simulink model "Simulation_BlackBox"  (R2022b)
settings: Solver=VariableStepAuto  StartTime=0.0  StopTime=100  RelTol=1e-3
undefined symbols (not defined in the file): DiscIntNeverNeededParam, drv, gbox, mot, sens, Tc, Ts
settings Model: Creator=Matteo  LastModifiedBy=david
settings SolverCC: AlgebraicLoopSolver=LineSearch
settings DebuggingCC: UnconnectedInputMsg=warning  UnconnectedOutputMsg=warning  UnconnectedLineMsg=warning  SFMachineParentedDataDiag=warning  ArithmeticOperatorsInVariantConditions=warning
settings ModelReferenceCC: EnableRefExpFcnMdlSchedulingChecks=on
settings SFSimCC: SimUseLocalCustomCode=off  CustomCodeUndefinedFunction=UseInterfaceOnly
settings RTWCC: RTWUseLocalCustomCode=off

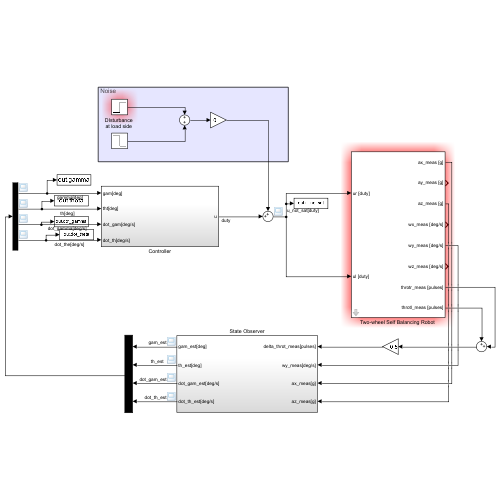
[thumbnail: Simulink's stored preview of the top-level diagram]
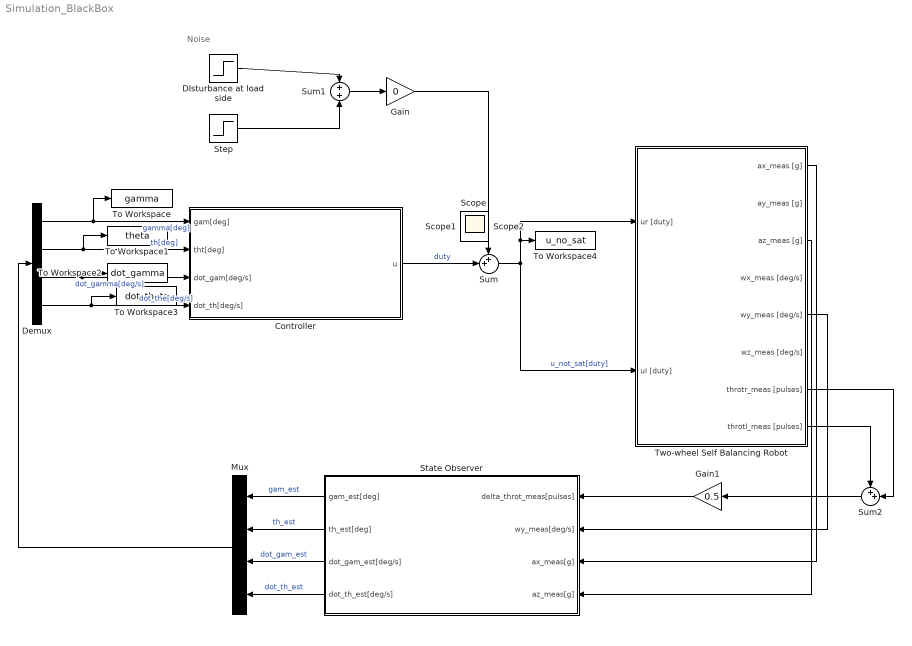
== system Simulation_BlackBox ==
  note: Noise
  Controller : Subsystem
  "DIsturbance at load side " : Step  Time=30  After=100  SampleTime=Ts
  Demux : Demux
  Gain : Gain  Gain=0
  Gain1 : Gain  Gain=0.5
  Mux : Mux
  State Observer : Subsystem
  Step : Step  Time=60  After=-100  SampleTime=0
  Sum : Sum  Inputs=++|
  Sum1 : Sum
  Sum2 : Sum  Inputs=++|
  To Workspace : ToWorkspace  VariableName=gamma  SaveFormat=Structure With Time  SampleTime=0.01
  To Workspace1 : ToWorkspace  VariableName=theta  SaveFormat=Structure With Time  SampleTime=0.01
  To Workspace2 : ToWorkspace  VariableName=dot_gamma  SaveFormat=Structure With Time  SampleTime=0.01
  To Workspace3 : ToWorkspace  VariableName=dot_theta  SaveFormat=Structure With Time  SampleTime=0.01
  To Workspace4 : ToWorkspace  VariableName=u_no_sat  SaveFormat=Structure With Time  SampleTime=0.01
  "Two-wheel Self Balancing Robot " : Subsystem  mask(Balancing robot (longitudinal + lateral dynamics)){initState=[0, 0, pi/36, 0, 0, 0], Ts=Ts}
      mask prompts: initState "Initial state [gam(0), psi(0), th(0), dot_gam(0), dot_psi(0), dot_th(0)]'"; Ts "Sample time:"
      mask help:
      | Balancing robot dynamic model.
      | Includes both the longitudinal and lateral (yaw) dynamics.
      mask init:
      | %% General parameters and conversion gains
      | 
      | %   gravity acc [m/s^2]
      | g = 9.81;
      | 
      | %   conversion gains
      | rpm2rads = 2*pi/60;         %   [rpm]   -> [rad/s]
      | rads2rpm = 60/2/pi;         %   [rad/s] -> [rpm]
      | rpm2degs = 360/60;          %   [rpm]   -> [deg/s]
      | degs2rpm = 60/360;          %   [deg/s] -> [rpm]
      | deg2rad = pi/180;           %   [deg]   -> [rad]
      | rad2deg = 180/pi;           %   [rad]   -> [deg]
      | g2ms2 = g;                  %   [acc_g] -> [m/s^2]
      | ms22g = 1/g;                %   [m/s^2] -> [acc_g]
      | ozin2Nm = 0.706e-2;         %   [oz*inch] -> [N*m]
      | 
      | 
      | %%  Battery data
      | 
      | %   electrical data
      | batt.UN = 11.1;     %   nominal voltage
      | 
      | 
      | %%  H-bridge PWM voltage driver
      | 
      | drv.Vbus = batt.UN;                     %   H-bridge DC bus voltage  
      | drv.pwm.bits = 8;                       %   PWM resolution [bits]
      | drv.pwm.levels = 2^drv.pwm.bits;        %   PWM levels
      | drv.pwm.Fs = 490;                       %   PWM frequency
      | drv.dutymax = drv.pwm.levels-1;         %   max duty cycle code
      | drv.duty2V = drv.Vbus/drv.dutymax;      %   duty cycle code (0-255) to voltage
      | drv.V2duty = drv.dutymax/drv.Vbus;      %   voltage to duty cycle code (0-255)
      | 
      | 
      | %%  Gearbox data 
      | 
      | gbox.N = 30;            %   reduction ratio
      | 
      | 
      | %%  Sensors data - Hall-effect encoder
      | 
      | %   Hall-effect encoder
      | sens.enc.ppr = 16*4;    %   pulses per rotation at motor side (w/ quadrature decoding)
      | sens.enc.pulse2deg = 360/sens.enc.ppr;
      | sens.enc.pulse2rad = 2*pi/sens.enc.ppr;
      | sens.enc.deg2pulse = sens.enc.ppr/360;
      | sens.enc.rad2pulse = sens.enc.ppr/2/pi;
      | 
      | 
      | %%  Sensors data - MPU6050 (accelerometer + gyro)
      | 
      | %   center of mass (CoM) position
      | sens.mpu.xb = 0;
      | sens.mpu.yb = 0;
      | sens.mpu.zb = 13.5e-3;
      | 
      | %       MPU6050 embedded accelerometer specs
      | sens.mpu.acc.bits = 16;
      | sens.mpu.acc.fs_g = 16;                                                         %   full-scale in "g" units
      | sens.mpu.acc.fs = sens.mpu.acc.fs_g * g2ms2;                                    %   full-scale in [m/s^2] 
      | sens.mpu.acc.g2LSB = floor(2^(sens.mpu.acc.bits-1)/sens.mpu.acc.fs_g);          %   sensitivity [LSB/g]
      | sens.mpu.acc.ms22LSB = sens.mpu.acc.g2LSB * ms22g;                              %   sensitvity [LSB/(m/s^2)]
      | sens.mpu.acc.LSB2g = sens.mpu.acc.fs_g/2^(sens.mpu.acc.bits-1);                 %   output quantization step [g/LSB]
      | sens.mpu.acc.LSB2ms2 = sens.mpu.acc.LSB2g * g2ms2;                              %   output quantization step [ms2/LSB]
      | sens.mpu.acc.bw = 94;                                                           %   output low-pass filter bandwidth
      | sens.mpu.acc.noisestd = 400e-6*sqrt(100);                                       %   output noise std [g-rms]
      | sens.mpu.acc.noisevar = sens.mpu.acc.noisestd^2;                                %   output noise var [g^2]
      | 
      | %       MPU6050 embdedded gyroscope specs
      | sens.mpu.gyro.bits = 16;
      | sens.mpu.gyro.fs_degs = 250;                                                    %   full scale in [deg/s (dps)]
      | sens.mpu.gyro.fs = sens.mpu.gyro.fs_degs * deg2rad;                             %   full scale in [rad/s]
      | sens.mpu.gyro.degs2LSB = floor(2^(sens.mpu.gyro.bits-1)/sens.mpu.gyro.fs_degs);	%   sensitivity [LSB/degs]
      | sens.mpu.gyro.rads2LSB = sens.mpu.gyro.degs2LSB * rad2deg;                      %   sensitivity [LSB/rads] 
      | sens.mpu.gyro.LSB2degs = sens.mpu.gyro.fs_degs/2^(sens.mpu.gyro.bits-1);        %   output quantization step [degs/LSB]
      | sens.mpu.gyro.LSB2rads = sens.mpu.gyro.LSB2degs * deg2rad;                      %   output quantization step [rads/LSB]
      | sens.mpu.gyro.bw = 98;                                                          %   output low-pass filter bandwidth
      | sens.mpu.gyro.noisestd = 5e-3*sqrt(100);                                        %   output noise std [degs-rms]
      | sens.mpu.gyro.noisevar = sens.mpu.acc.noisestd ^2;                              %   output noise var [degs^2]
      mask Help:
      | Riccardo Antonello (antonello@dei.unipd.it)
      | 
      | May 19, 2020
      | 
      | Dept. of Information Engineering, University of Padova
  Scope : Scope
  Scope1 : Scope
  Scope2 : Scope
  wires:
  "DIsturbance at load side "/1 -> Sum1/1
  Sum2/1 -> Gain1/1
  "Two-wheel Self Balancing Robot "/5(wy_meas [deg/s]) -> State Observer/2(wy_meas[deg/s])
  "Two-wheel Self Balancing Robot "/1(ax_meas [g]) -> State Observer/3(ax_meas[g])
  "Two-wheel Self Balancing Robot "/3(az_meas [g]) -> State Observer/4(az_meas[g])
  Sum/1 -> "Two-wheel Self Balancing Robot "/1(ur [duty]), To Workspace4/1, "Two-wheel Self Balancing Robot "/2(ul [duty])  "u_not_sat[duty]"
  Controller/1(u) -> Sum/2  "duty"
  Demux/3 -> To Workspace2/1, Controller/3(dot_gam[deg/s])  "dot_gamma[deg/s]"
  Demux/2 -> To Workspace1/1, Controller/2(tht[deg])  "th[deg]"
  Demux/1 -> To Workspace/1, Controller/1(gam[deg])  "gamma[deg]"
  Demux/4 -> To Workspace3/1, Controller/4(dot_th[deg/s])  "dot_the[deg/s]"
  State Observer/1(gam_est[deg]) -> Mux/1  "gam_est"
  State Observer/2(th_est[deg]) -> Mux/2  "th_est"
  State Observer/3(dot_gam_est[deg/s]) -> Mux/3  "dot_gam_est"
  State Observer/4(dot_th_est[deg/s]) -> Mux/4  "dot_th_est"
  Mux/1 -> Demux/1
  Sum1/1 -> Gain/1
  Step/1 -> Sum1/2
  Gain/1 -> Sum/1
  Gain1/1 -> State Observer/1(delta_throt_meas[pulses])
  "Two-wheel Self Balancing Robot "/7(throtr_meas [pulses]) -> Sum2/2
  "Two-wheel Self Balancing Robot "/8(throtl_meas [pulses]) -> Sum2/1

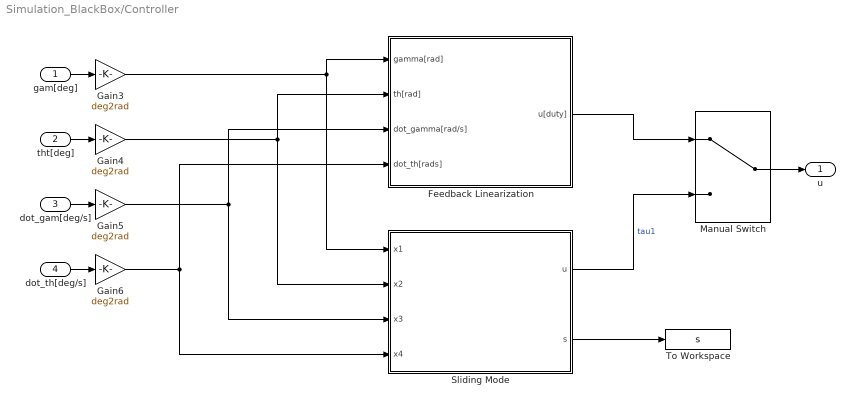
== system Simulation_BlackBox/Controller ==
  gam[deg] : Inport
  tht[deg] : Inport  Port=2
  dot_gam[deg/s] : Inport  Port=3
  dot_th[deg/s] : Inport  Port=4
  Feedback Linearization : Subsystem
  Gain{3..6} (4 alike) : Gain  Gain=deg2rad
  Manual Switch : ManualSwitch
  Sliding Mode : MATLAB Function  TreatAsAtomicUnit=on
  To Workspace : ToWorkspace  VariableName=s  SaveFormat=Structure With Time  SampleTime=0.01
  u : Outport  VectorParamsAs1DForOutWhenUnconnected=off
  wires:
  gam[deg]/1 -> Gain3/1
  dot_th[deg/s]/1 -> Gain6/1
  dot_gam[deg/s]/1 -> Gain5/1
  tht[deg]/1 -> Gain4/1
  Gain3/1 -> Feedback Linearization/1(gamma[rad]), Sliding Mode/1(x1)
  Gain4/1 -> Feedback Linearization/2(th[rad]), Sliding Mode/2(x2)
  Gain5/1 -> Feedback Linearization/3(dot_gamma[rad/s]), Sliding Mode/3(x3)
  Gain6/1 -> Feedback Linearization/4(dot_th[rads]), Sliding Mode/4(x4)
  Sliding Mode/1(u) -> Manual Switch/2  "tau1"
  Sliding Mode/2(s) -> To Workspace/1
  Manual Switch/1 -> u/1
  Feedback Linearization/1(u[duty]) -> Manual Switch/1

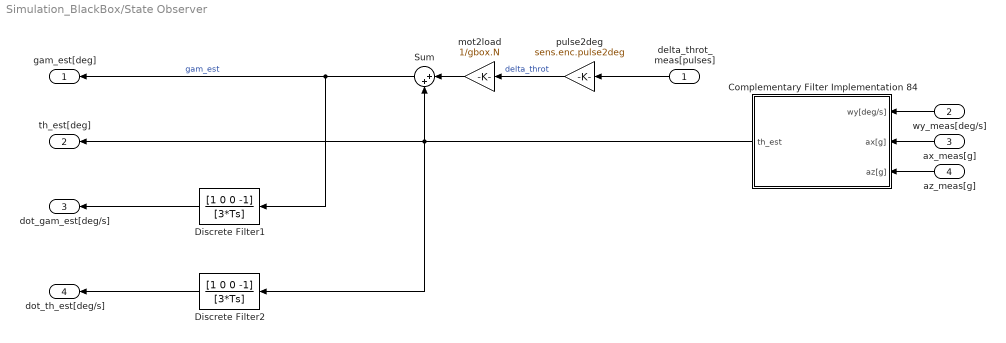
== system Simulation_BlackBox/State Observer ==
  delta_throt_meas[pulses] : Inport
  wy_meas[deg/s] : Inport  Port=2
  ax_meas[g] : Inport  Port=3
  az_meas[g] : Inport  Port=4
  Complementary Filter Implementation 84 : Subsystem
  Discrete Filter1 : DiscreteFilter  Numerator=[1 0 0 -1]  Denominator=[3*Ts]  SampleTime=Ts
  Discrete Filter2 : DiscreteFilter  Numerator=[1 0 0 -1]  Denominator=[3*Ts]  SampleTime=Ts
  Sum : Sum  Inputs=|++
  mot2load : Gain  Gain=1/gbox.N
  pulse2deg : Gain  Gain=sens.enc.pulse2deg
  gam_est[deg] : Outport  VectorParamsAs1DForOutWhenUnconnected=off
  th_est[deg] : Outport  Port=2  VectorParamsAs1DForOutWhenUnconnected=off
  dot_gam_est[deg/s] : Outport  Port=3  VectorParamsAs1DForOutWhenUnconnected=off
  dot_th_est[deg/s] : Outport  Port=4  VectorParamsAs1DForOutWhenUnconnected=off
  wires:
  Sum/1 -> Discrete Filter1/1, gam_est[deg]/1  "gam_est"
  Discrete Filter2/1 -> dot_th_est[deg/s]/1
  mot2load/1 -> Sum/1
  delta_throt_meas[pulses]/1 -> pulse2deg/1
  Complementary Filter Implementation 84/1(th_est) -> Discrete Filter2/1, th_est[deg]/1, Sum/2
  pulse2deg/1 -> mot2load/1  "delta_throt"
  Discrete Filter1/1 -> dot_gam_est[deg/s]/1
  az_meas[g]/1 -> Complementary Filter Implementation 84/3(az[g])
  ax_meas[g]/1 -> Complementary Filter Implementation 84/2(ax[g])
  wy_meas[deg/s]/1 -> Complementary Filter Implementation 84/1(wy[deg/s])

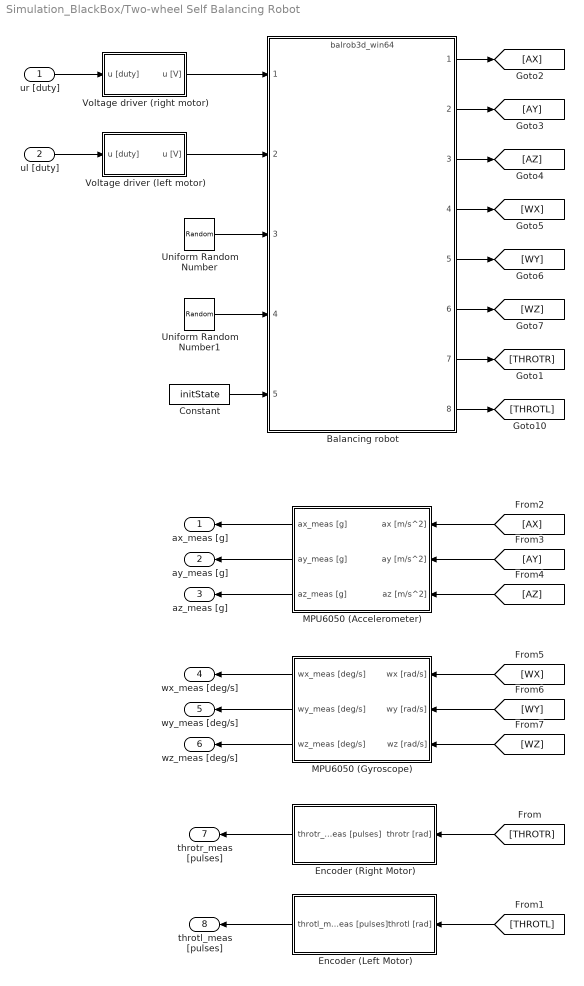
== system Simulation_BlackBox/Two-wheel Self Balancing Robot  ==
  ur [duty] : Inport
  ul [duty] : Inport  Port=2
  Balancing robot : ModelReference  ModelNameDialog=balrob3d_win64.slxp  ModelReferenceVersion=1.741  CopyOfModelProtected=on
  Constant : Constant  Value=initState
  Encoder (Left Motor) : Subsystem
  Encoder (Right Motor) : Subsystem
  MPU6050 (Accelerometer) : Subsystem
  MPU6050 (Gyroscope) : Subsystem
  Uniform Random Number : UniformRandomNumber  Minimum=0.7  Maximum=1.3  SampleTime=1
  Uniform Random Number1 : UniformRandomNumber  Minimum=0.7  Maximum=1.3  Seed=10  SampleTime=1
  Voltage driver (left motor) : Subsystem
  Voltage driver (right motor) : Subsystem
  ax_meas [g] : Outport
  ay_meas [g] : Outport  Port=2
  az_meas [g] : Outport  Port=3
  wx_meas [deg/s] : Outport  Port=4
  wy_meas [deg/s] : Outport  Port=5
  wz_meas [deg/s] : Outport  Port=6
  throtr_meas [pulses] : Outport  Port=7
  throtl_meas [pulses] : Outport  Port=8
  wires:
  ur [duty]/1 -> Voltage driver (right motor)/1(u [duty])
  [WX] -> MPU6050 (Gyroscope)/1(wx [rad/s])
  Balancing robot/2 -> [AY]
  Balancing robot/4 -> [WX]
  Balancing robot/8 -> [THROTL]
  Balancing robot/1 -> [AX]
  [THROTL] -> Encoder (Left Motor)/1(throtl [rad])
  Balancing robot/6 -> [WZ]
  Balancing robot/7 -> [THROTR]
  Balancing robot/5 -> [WY]
  [AX] -> MPU6050 (Accelerometer)/1(ax [m/s^2])
  [WY] -> MPU6050 (Gyroscope)/2(wy [rad/s])
  Balancing robot/3 -> [AZ]
  [WZ] -> MPU6050 (Gyroscope)/3(wz [rad/s])
  [AZ] -> MPU6050 (Accelerometer)/3(az [m/s^2])
  [THROTR] -> Encoder (Right Motor)/1(throtr [rad])
  ul [duty]/1 -> Voltage driver (left motor)/1(u [duty])
  [AY] -> MPU6050 (Accelerometer)/2(ay [m/s^2])
  MPU6050 (Accelerometer)/1(ax_meas [g]) -> ax_meas [g]/1
  MPU6050 (Accelerometer)/2(ay_meas [g]) -> ay_meas [g]/1
  MPU6050 (Accelerometer)/3(az_meas [g]) -> az_meas [g]/1
  MPU6050 (Gyroscope)/1(wx_meas [deg/s]) -> wx_meas [deg/s]/1
  MPU6050 (Gyroscope)/2(wy_meas [deg/s]) -> wy_meas [deg/s]/1
  MPU6050 (Gyroscope)/3(wz_meas [deg/s]) -> wz_meas [deg/s]/1
  Encoder (Right Motor)/1(throtr_meas [pulses]) -> throtr_meas [pulses]/1
  Encoder (Left Motor)/1(throtl_meas [pulses]) -> throtl_meas [pulses]/1
  Voltage driver (right motor)/1(u [V]) -> Balancing robot/1
  Voltage driver (left motor)/1(u [V]) -> Balancing robot/2
  Uniform Random Number/1 -> Balancing robot/3
  Uniform Random Number1/1 -> Balancing robot/4
  Constant/1 -> Balancing robot/5

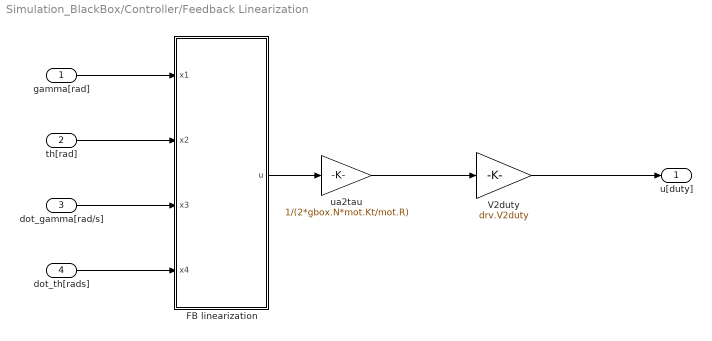
== system Simulation_BlackBox/Controller/Feedback Linearization ==
  gamma[rad] : Inport
  th[rad] : Inport  Port=2
  dot_gamma[rad/s] : Inport  Port=3
  dot_th[rads] : Inport  Port=4
  FB linearization : MATLAB Function  TreatAsAtomicUnit=on
  V2duty : Gain  Gain=drv.V2duty
  ua2tau : Gain  Gain=1/(2*gbox.N*mot.Kt/mot.R)
  u[duty] : Outport
  wires:
  FB linearization/1(u) -> ua2tau/1
  dot_th[rads]/1 -> FB linearization/4(x4)
  th[rad]/1 -> FB linearization/2(x2)
  gamma[rad]/1 -> FB linearization/1(x1)
  dot_gamma[rad/s]/1 -> FB linearization/3(x3)
  ua2tau/1 -> V2duty/1
  V2duty/1 -> u[duty]/1

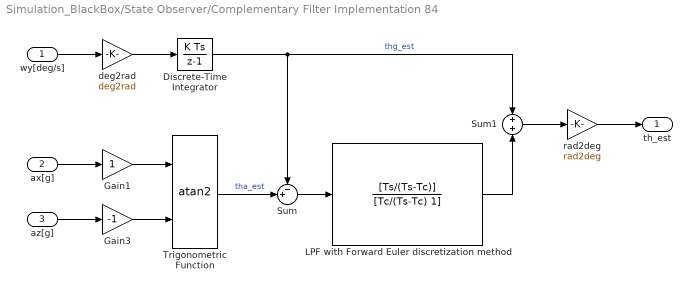
== system Simulation_BlackBox/State Observer/Complementary Filter Implementation 84 ==
  wy[deg/s] : Inport
  ax[g] : Inport  Port=2
  az[g] : Inport  Port=3
  Discrete-Time Integrator : DiscreteIntegrator  SampleTime=Ts  ICPrevOutput=DiscIntNeverNeededParam  ICPrevScaledInput=DiscIntNeverNeededParam
  Gain1 : Gain
  Gain3 : Gain  Gain=-1
  LPF with Forward Euler discretization method : DiscreteTransferFcn  Numerator=[Ts/(Ts-Tc)]  Denominator=[Tc/(Ts-Tc) 1]  SampleTime=Ts
  Sum : Sum  Inputs=-+|
  Sum1 : Sum  Inputs=+|+
  Trigonometric Function : Trigonometry  Operator=atan2
  deg2rad : Gain  Gain=deg2rad
  rad2deg : Gain  Gain=rad2deg
  th_est : Outport  VectorParamsAs1DForOutWhenUnconnected=off
  wires:
  Gain3/1 -> Trigonometric Function/2
  Trigonometric Function/1 -> Sum/2  "tha_est"
  az[g]/1 -> Gain3/1
  Gain1/1 -> Trigonometric Function/1
  Discrete-Time Integrator/1 -> Sum1/1, Sum/1  "thg_est"
  deg2rad/1 -> Discrete-Time Integrator/1
  Sum1/1 -> rad2deg/1
  wy[deg/s]/1 -> deg2rad/1
  ax[g]/1 -> Gain1/1
  LPF with Forward Euler discretization method/1 -> Sum1/2
  Sum/1 -> LPF with Forward Euler discretization method/1
  rad2deg/1 -> th_est/1

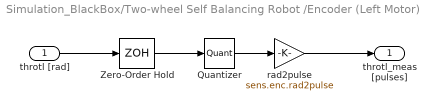
== system Simulation_BlackBox/Two-wheel Self Balancing Robot /Encoder (Left Motor) ==
  throtl [rad] : Inport
  Quantizer : Quantizer  QuantizationInterval=sens.enc.pulse2rad
  Zero-Order Hold : ZeroOrderHold  SampleTime=Ts
  rad2pulse : Gain  Gain=sens.enc.rad2pulse
  throtl_meas [pulses] : Outport
  wires:
  Quantizer/1 -> rad2pulse/1
  Zero-Order Hold/1 -> Quantizer/1
  throtl [rad]/1 -> Zero-Order Hold/1
  rad2pulse/1 -> throtl_meas [pulses]/1

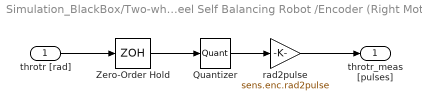
== system Simulation_BlackBox/Two-wheel Self Balancing Robot /Encoder (Right Motor) ==
  throtr [rad] : Inport
  Quantizer : Quantizer  QuantizationInterval=sens.enc.pulse2rad
  Zero-Order Hold : ZeroOrderHold  SampleTime=Ts
  rad2pulse : Gain  Gain=sens.enc.rad2pulse
  throtr_meas [pulses] : Outport
  wires:
  throtr [rad]/1 -> Zero-Order Hold/1
  Zero-Order Hold/1 -> Quantizer/1
  Quantizer/1 -> rad2pulse/1
  rad2pulse/1 -> throtr_meas [pulses]/1

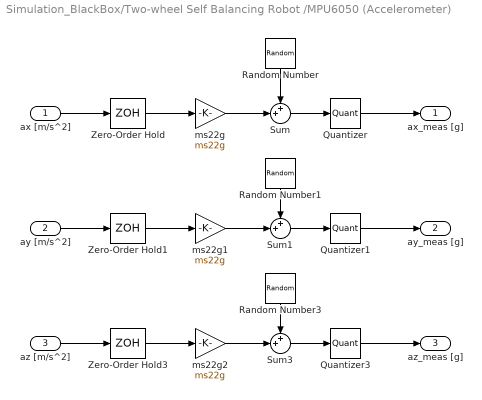
== system Simulation_BlackBox/Two-wheel Self Balancing Robot /MPU6050 (Accelerometer) ==
  ax [m/s^2] : Inport
  ay [m/s^2] : Inport  Port=2
  az [m/s^2] : Inport  Port=3
  Quantizer : Quantizer  QuantizationInterval=sens.mpu.acc.LSB2g
  Quantizer1 : Quantizer  QuantizationInterval=sens.mpu.acc.LSB2g
  Quantizer3 : Quantizer  QuantizationInterval=sens.mpu.acc.LSB2g
  Random Number : RandomNumber  Variance=sens.mpu.acc.noisevar  Seed=1  SampleTime=Ts
  Random Number1 : RandomNumber  Variance=sens.mpu.acc.noisevar  Seed=10  SampleTime=Ts
  Random Number3 : RandomNumber  Variance=sens.mpu.acc.noisevar  Seed=100  SampleTime=Ts
  Sum : Sum  Inputs=++|
  Sum1 : Sum  Inputs=++|
  Sum3 : Sum  Inputs=++|
  Zero-Order Hold : ZeroOrderHold  SampleTime=Ts
  Zero-Order Hold1 : ZeroOrderHold  SampleTime=Ts
  Zero-Order Hold3 : ZeroOrderHold  SampleTime=Ts
  ms22g : Gain  Gain=ms22g
  ms22g1 : Gain  Gain=ms22g
  ms22g2 : Gain  Gain=ms22g
  ax_meas [g] : Outport
  ay_meas [g] : Outport  Port=2
  az_meas [g] : Outport  Port=3
  wires:
  ax [m/s^2]/1 -> Zero-Order Hold/1
  Zero-Order Hold1/1 -> ms22g1/1
  Sum1/1 -> Quantizer1/1
  ms22g/1 -> Sum/2
  ay [m/s^2]/1 -> Zero-Order Hold1/1
  Sum3/1 -> Quantizer3/1
  ms22g1/1 -> Sum1/2
  Random Number1/1 -> Sum1/1
  Random Number/1 -> Sum/1
  Sum/1 -> Quantizer/1
  Random Number3/1 -> Sum3/1
  ms22g2/1 -> Sum3/2
  Zero-Order Hold3/1 -> ms22g2/1
  az [m/s^2]/1 -> Zero-Order Hold3/1
  Zero-Order Hold/1 -> ms22g/1
  Quantizer/1 -> ax_meas [g]/1
  Quantizer1/1 -> ay_meas [g]/1
  Quantizer3/1 -> az_meas [g]/1

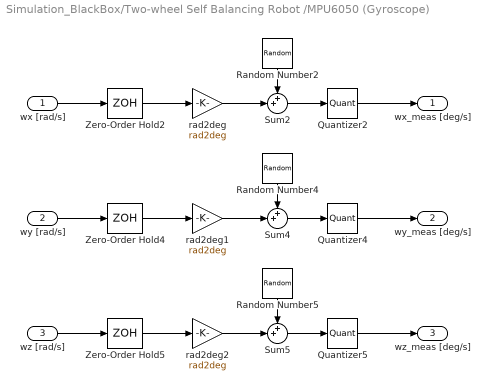
== system Simulation_BlackBox/Two-wheel Self Balancing Robot /MPU6050 (Gyroscope) ==
  wx [rad/s] : Inport
  wy [rad/s] : Inport  Port=2
  wz [rad/s] : Inport  Port=3
  Quantizer2 : Quantizer  QuantizationInterval=sens.mpu.gyro.LSB2degs
  Quantizer4 : Quantizer  QuantizationInterval=sens.mpu.gyro.LSB2degs
  Quantizer5 : Quantizer  QuantizationInterval=sens.mpu.gyro.LSB2degs
  Random Number2 : RandomNumber  Variance=sens.mpu.gyro.noisevar  Seed=2  SampleTime=Ts
  Random Number4 : RandomNumber  Variance=sens.mpu.gyro.noisevar  Seed=20  SampleTime=Ts
  Random Number5 : RandomNumber  Variance=sens.mpu.gyro.noisevar  Seed=200  SampleTime=Ts
  Sum2 : Sum  Inputs=++|
  Sum4 : Sum  Inputs=++|
  Sum5 : Sum  Inputs=++|
  Zero-Order Hold2 : ZeroOrderHold  SampleTime=Ts
  Zero-Order Hold4 : ZeroOrderHold  SampleTime=Ts
  Zero-Order Hold5 : ZeroOrderHold  SampleTime=Ts
  rad2deg : Gain  Gain=rad2deg
  rad2deg1 : Gain  Gain=rad2deg
  rad2deg2 : Gain  Gain=rad2deg
  wx_meas [deg/s] : Outport
  wy_meas [deg/s] : Outport  Port=2
  wz_meas [deg/s] : Outport  Port=3
  wires:
  Random Number2/1 -> Sum2/1
  Sum2/1 -> Quantizer2/1
  Quantizer2/1 -> wx_meas [deg/s]/1
  Zero-Order Hold5/1 -> rad2deg2/1
  Sum4/1 -> Quantizer4/1
  rad2deg/1 -> Sum2/2
  rad2deg2/1 -> Sum5/2
  Random Number5/1 -> Sum5/1
  Zero-Order Hold4/1 -> rad2deg1/1
  Sum5/1 -> Quantizer5/1
  Random Number4/1 -> Sum4/1
  Zero-Order Hold2/1 -> rad2deg/1
  Quantizer5/1 -> wz_meas [deg/s]/1
  wz [rad/s]/1 -> Zero-Order Hold5/1
  wx [rad/s]/1 -> Zero-Order Hold2/1
  rad2deg1/1 -> Sum4/2
  Quantizer4/1 -> wy_meas [deg/s]/1
  wy [rad/s]/1 -> Zero-Order Hold4/1

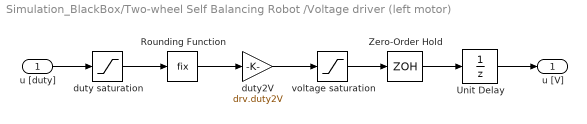
== system Simulation_BlackBox/Two-wheel Self Balancing Robot /Voltage driver (left motor) ==
  u [duty] : Inport
  Rounding Function : Rounding  Operator=fix
  Unit Delay : UnitDelay  SampleTime=1/drv.pwm.Fs  HasFrameUpgradeWarning=on
  Zero-Order Hold : ZeroOrderHold  SampleTime=Ts
  duty saturation : Saturate  UpperLimit=255  LowerLimit=-255
  duty2V : Gain  Gain=drv.duty2V
  voltage saturation : Saturate  UpperLimit=drv.Vbus  LowerLimit=-drv.Vbus
  u [V] : Outport
  wires:
  Zero-Order Hold/1 -> Unit Delay/1
  u [duty]/1 -> duty saturation/1
  voltage saturation/1 -> Zero-Order Hold/1
  duty saturation/1 -> Rounding Function/1
  Rounding Function/1 -> duty2V/1
  duty2V/1 -> voltage saturation/1
  Unit Delay/1 -> u [V]/1

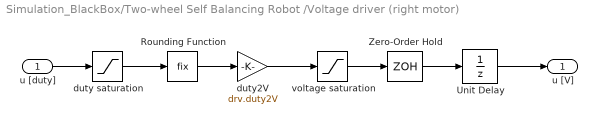
== system Simulation_BlackBox/Two-wheel Self Balancing Robot /Voltage driver (right motor) ==
  u [duty] : Inport
  Rounding Function : Rounding  Operator=fix
  Unit Delay : UnitDelay  SampleTime=1/drv.pwm.Fs  HasFrameUpgradeWarning=on
  Zero-Order Hold : ZeroOrderHold  SampleTime=Ts
  duty saturation : Saturate  UpperLimit=255  LowerLimit=-255
  duty2V : Gain  Gain=drv.duty2V
  voltage saturation : Saturate  UpperLimit=drv.Vbus  LowerLimit=-drv.Vbus
  u [V] : Outport
  wires:
  u [duty]/1 -> duty saturation/1
  duty saturation/1 -> Rounding Function/1
  Zero-Order Hold/1 -> Unit Delay/1
  voltage saturation/1 -> Zero-Order Hold/1
  Rounding Function/1 -> duty2V/1
  duty2V/1 -> voltage saturation/1
  Unit Delay/1 -> u [V]/1

== matlab function Simulation_BlackBox/Controller/Feedback Linearization/FB linearization ==
  data: x1 input; x2 input; u output; x3 input; x4 input; num1 parameter
function u   = fcn(x1, x2, x3 ,x4, num1)

f=[x3;
    x4;
    -(num1.g2*num1.m12*sin(x2) - num1.f11*num1.m22*x3 + num1.f21*num1.m12*x3 + num1.f22*num1.m12*x4 - num1.f21*num1.m22*x4 + num1.f21*num1.k*x3*cos(x2) + num1.f22*num1.k*x4*cos(x2) - num1.c12*num1.m22*x4^2*sin(x2) + num1.g2*num1.k*cos(x2)*sin(x2))/(num1.k^2*cos(x2)^2 + 2*num1.k*num1.m12*cos(x2) + num1.m12^2 - num1.m11*num1.m22);
    -(num1.f11*num1.m12*x3 - num1.g2*num1.m11*sin(x2) - num1.f21*num1.m11*x3 + num1.f21*num1.m12*x4 - num1.f22*num1.m11*x4 + num1.f11*num1.k*x3*cos(x2) + num1.f21*num1.k*x4*cos(x2) + num1.c12*num1.m12*x4^2*sin(x2) + num1.c12*num1.k*x4^2*cos(x2)*sin(x2))/(num1.k^2*cos(x2)^2 + 2*num1.k*num1.m12*cos(x2) + num1.m12^2 - num1.m11*num1.m22)];
g=[0; 0;
    -(num1.m12 + num1.m22 + num1.k*cos(x2))/(num1.k^2*cos(x2)^2 + 2*num1.k*num1.m12*cos(x2) + num1.m12^2 - num1.m11*num1.m22);
    (num1.m11 + num1.m12 + num1.k*cos(x2))/(num1.k^2*cos(x2)^2 + 2*num1.k*num1.m12*cos(x2) + num1.m12^2 - num1.m11*num1.m22)];

%K= [72 17];
K=[100.25, 20];
x1_d=pi/18;
c= [10 1 15];
v =-K(1)*(x2)-K(2)*x4;
u=(-f(4)+v)/g(4)-((-c(1)*(x1-x1_d)-c(3)*x3-c(2)*f(3))*g(4)-c(2)*g(3)*(v-f(4)))/(c(2)*g(3)*g(4));
%u=(-f(4)+v)/g(4);
end

== matlab function Simulation_BlackBox/Controller/Sliding Mode ==
  data: x1 input; x2 input; u output; x3 input; x4 input; s output
function [u,s]  = fcn(x1, x2, x3 ,x4)


K=200;
%K=5;
s = x4+K*x2;
a=1;
if(abs(s)>a)
    sat= sign(s);
else
    sat=s/a;
end

u =255*sat;
%u=255*sign(s);


end
